simulink model "sampleModel1534"  (R2023a)
settings: Solver=VariableStepAuto  StartTime=0.0  StopTime=10.0  RelTol=1e-3
libraries: hdlsllib x7, simulink x1
settings Model: Creator=user1  LastModifiedBy=user1

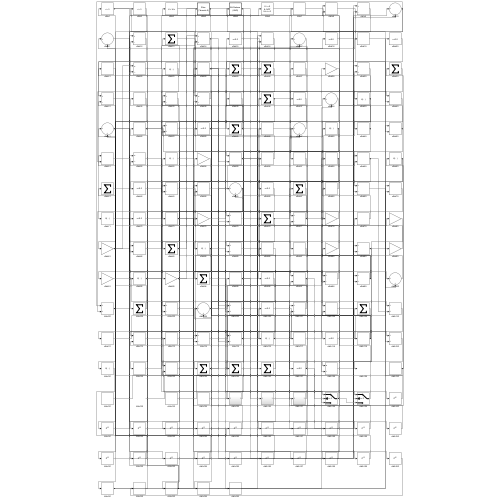
[thumbnail: Simulink's stored preview of the top-level diagram]
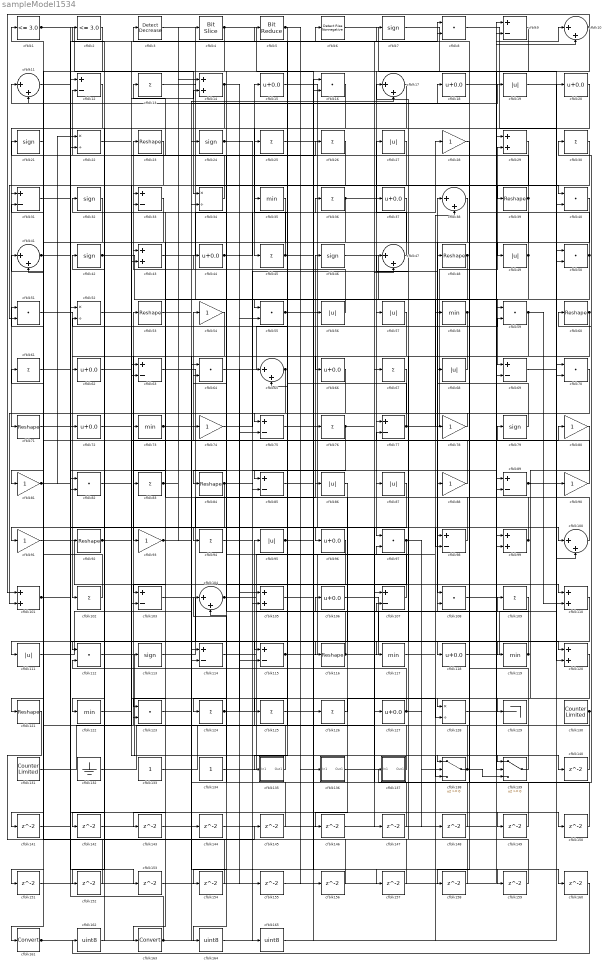
== system sampleModel1534 ==
  cfblk1 : hdlsllib/Logic and Bit Operations/Compare To Constant  relop=<=  const=3.0  OutDataTypeStr=boolean
  cfblk{10..11,17,38,41,47,65,100,104} (9 alike) : Sum  Inputs=|++
  cfblk{14,29,43,99,101,105,110,120} (8 alike) : Sum
  cfblk{13,25..26,30,36,45,61,67,76,83,94,102,109,124..126} (16 alike) : Sum  Inputs=+
  cfblk{9,12,31,33,63,69,75,77,85,89,98,103,107,114..115} (15 alike) : Sum  Inputs=+-
  cfblk{15,18,20,37,44,62,66,72,96,106,118,127} (12 alike) : Bias  Bias=0.0  SaturateOnIntegerOverflow=off
  cfblk{8,16,40,50..51,55,59,64,70,82,97,108,112,123} (14 alike) : DotProduct  OutDataTypeStr=Inherit: Inherit via internal rule
  cfblk{19,27,49,56..57,68,86..87,95,111} (10 alike) : Abs  SaturateOnIntegerOverflow=off
  cfblk{7,21,24,32,42,46,79,113} (8 alike) : Signum
  cfblk{23,39,48,53,60,71,84,92,116,121} (10 alike) : Reshape
  cfblk{35,58,73,117,119,122} (6 alike) : MinMax
  cfblk{22,34,52,128} (4 alike) : Product  Inputs=*/  RndMeth=Zero  SaturateOnIntegerOverflow=on
  cfblk129 : Terminator
  cfblk130 : hdlsllib/Sources/Counter Limited  uplimit=7  tsamp=-1
  cfblk131 : hdlsllib/Sources/Counter Limited  uplimit=7  tsamp=-1
  cfblk132 : Ground
  cfblk133 : Constant  SampleTime=-1
  cfblk134 : Constant  SampleTime=-1
  cfblk135 : Subsystem
      settings: LibrarySourceBlock=|
      | hdlsllib/Ports &
      | Subsystems/Subsystem
  cfblk136 : Subsystem
      settings: LibrarySourceBlock=|
      | hdlsllib/Ports &
      | Subsystems/Subsystem
  cfblk137 : Subsystem
      settings: LibrarySourceBlock=|
      | hdlsllib/Ports &
      | Subsystems/Subsystem
  cfblk138 : Switch  SaturateOnIntegerOverflow=off  InputSameDT=off
  cfblk139 : Switch  SaturateOnIntegerOverflow=off  InputSameDT=off
  cfblk{140..160} (21 alike) : Delay  SampleTime=1
  cfblk161 : DataTypeConversion  SaturateOnIntegerOverflow=off  RndMeth=Floor
  cfblk162 : DataTypeConversion  OutDataTypeStr=uint8  SaturateOnIntegerOverflow=off  RndMeth=Floor
  cfblk163 : DataTypeConversion  SaturateOnIntegerOverflow=off  RndMeth=Floor
  cfblk164 : DataTypeConversion  OutDataTypeStr=uint8  SaturateOnIntegerOverflow=off  RndMeth=Floor
  cfblk165 : DataTypeConversion  OutDataTypeStr=uint8  SaturateOnIntegerOverflow=off  RndMeth=Floor
  cfblk2 : hdlsllib/Logic and Bit Operations/Compare To Constant  relop=<=  const=3.0  OutDataTypeStr=boolean
  cfblk{28,54,74,78,80..81,88,90..91,93} (10 alike) : Gain
  cfblk3 : simulink/Logic and Bit Operations/Detect Decrease  vinit=0.0  OutDataTypeStr=boolean
      settings: LibrarySourceBlock=|
      | hdlsllib/Logic and Bit
      | Operations/Detect
      | Decrease
  cfblk4 : hdlsllib/Logic and Bit Operations/Bit Slice  lidx=7  ridx=0
  cfblk5 : hdlsllib/Logic and Bit Operations/Bit Reduce  mode=AND
  cfblk6 : hdlsllib/Logic and Bit Operations/Detect Rise Nonnegative  vinit=0  OutDataTypeStr=boolean
  wires:
  cfblk119/1 -> cfblk38/1, cfblk33/2, cfblk21/1
  cfblk63/1 -> cfblk96/1
  cfblk86/1 -> cfblk111/1
  cfblk14/1 -> cfblk71/1, cfblk115/2
  cfblk49/1 -> cfblk3/1, cfblk135/1(In1)
  cfblk10/1 -> cfblk101/1, cfblk22/2, cfblk154/1
  cfblk137/1(Out1) -> cfblk51/1
  cfblk17/1 -> cfblk45/1
  cfblk25/1 -> cfblk40/1
  cfblk88/1 -> cfblk54/1
  cfblk106/1 -> cfblk118/1
  cfblk39/1 -> cfblk108/1, cfblk13/1, cfblk103/2
  cfblk90/1 -> cfblk61/1
  cfblk78/1 -> cfblk75/1
  cfblk132/1 -> cfblk95/1
  cfblk70/1 -> cfblk163/1
  cfblk9/1 -> cfblk97/1
  cfblk66/1 -> cfblk101/2
  cfblk27/1 -> cfblk57/1
  cfblk15/1 -> cfblk127/1
  cfblk84/1 -> cfblk64/2, cfblk141/1, cfblk159/1
  cfblk114/1 -> cfblk109/1
  cfblk38/1 -> cfblk84/1
  cfblk60/1 -> cfblk102/1, cfblk117/1
  cfblk21/1 -> cfblk81/1
  cfblk55/1 -> cfblk98/1, cfblk89/2
  cfblk13/1 -> cfblk69/1
  cfblk89/1 -> cfblk128/1, cfblk100/2
  cfblk108/1 -> cfblk120/1
  cfblk136/1(Out1) -> cfblk30/1
  cfblk99/1 -> cfblk17/1, cfblk33/1, cfblk65/2
  cfblk45/1 -> cfblk15/1, cfblk149/1
  cfblk32/1 -> cfblk91/1
  cfblk34/1 -> cfblk12/2
  cfblk1/1 -> cfblk34/1, cfblk100/1
  cfblk36/1 -> cfblk121/1, cfblk8/1
  cfblk74/1 -> cfblk48/1
  cfblk53/1 -> cfblk17/2
  cfblk135/1(Out1) -> cfblk53/1
  cfblk113/1 -> cfblk46/1
  cfblk77/1 -> cfblk29/2, cfblk52/2
  cfblk101/1 -> cfblk41/1, cfblk153/1
  cfblk54/1 -> cfblk93/1
  cfblk59/1 -> cfblk77/1, cfblk110/2
  cfblk44/1 -> cfblk36/1, cfblk55/2
  cfblk30/1 -> cfblk69/2
  cfblk115/1 -> cfblk67/1, cfblk35/1
  cfblk43/1 -> cfblk28/1
  cfblk67/1 -> cfblk85/1
  cfblk134/1 -> cfblk106/1
  cfblk56/1 -> cfblk23/1
  cfblk127/1 -> cfblk112/2, cfblk148/1
  cfblk124/1 -> cfblk76/1, cfblk65/1
  cfblk109/1 -> cfblk107/2
  cfblk104/1 -> cfblk38/2, cfblk75/2
  cfblk3/1 -> cfblk39/1
  cfblk107/1 -> cfblk44/1
  cfblk8/1 -> cfblk40/2
  cfblk102/1 -> cfblk41/2
  cfblk52/1 -> cfblk128/2
  cfblk48/1 -> cfblk83/1, cfblk55/1
  cfblk19/1 -> cfblk90/1
  cfblk41/1 -> cfblk99/2, cfblk150/1
  cfblk83/1 -> cfblk43/1, cfblk14/1
  cfblk69/1 -> cfblk120/2
  cfblk79/1 -> cfblk68/1
  cfblk16/1 -> cfblk122/1
  cfblk5/1 -> cfblk125/1, cfblk156/1
  cfblk51/1 -> cfblk62/1
  cfblk117/1 -> cfblk79/1
  cfblk37/1 -> cfblk73/1
  cfblk47/1 -> cfblk27/1
  cfblk72/1 -> cfblk26/1
  cfblk111/1 -> cfblk18/1
  cfblk125/1 -> cfblk16/1
  cfblk42/1 -> cfblk85/2, cfblk14/2
  cfblk112/1 -> cfblk139/1
  cfblk95/1 -> cfblk19/1, cfblk136/1(In1)
  cfblk82/1 -> cfblk43/2
  cfblk118/1 -> cfblk20/1
  cfblk92/1 -> cfblk116/1, cfblk138/1
  cfblk85/1 -> cfblk16/2
  cfblk40/1 -> cfblk49/1
  cfblk65/1 -> cfblk103/1, cfblk152/1
  cfblk73/1 -> cfblk98/2, cfblk160/1
  cfblk58/1 -> cfblk123/1, cfblk114/2
  cfblk130/1 -> cfblk123/2, cfblk60/1
  cfblk26/1 -> cfblk51/2
  cfblk24/1 -> cfblk138/3, cfblk105/1, cfblk155/1
  cfblk6/1 -> cfblk139/2
  cfblk91/1 -> cfblk137/1(In1)
  cfblk138/1 -> cfblk139/3, cfblk5/1
  cfblk139/1 -> cfblk108/2
  cfblk131/1 -> cfblk63/1
  cfblk76/1 -> cfblk37/1, cfblk105/2
  cfblk2/1 -> cfblk161/1
  cfblk46/1 -> cfblk78/1
  cfblk20/1 -> cfblk25/1
  cfblk80/1 -> cfblk129/1
  cfblk50/1 -> cfblk11/2, cfblk115/1
  cfblk126/1 -> cfblk86/1
  cfblk81/1 -> cfblk72/1, cfblk22/1
  cfblk18/1 -> cfblk10/1
  cfblk87/1 -> cfblk94/1
  cfblk100/1 -> cfblk88/1
  cfblk116/1 -> cfblk32/1, cfblk9/2
  cfblk98/1 -> cfblk47/1
  cfblk94/1 -> cfblk110/1
  cfblk68/1 -> cfblk66/1
  cfblk128/1 -> cfblk10/2
  cfblk93/1 -> cfblk24/1, cfblk4/1
  cfblk57/1 -> cfblk112/1
  cfblk22/1 -> cfblk6/1
  cfblk61/1 -> cfblk119/1
  cfblk4/1 -> cfblk126/1, cfblk82/2
  cfblk23/1 -> cfblk63/2
  cfblk97/1 -> cfblk104/2, cfblk138/2
  cfblk62/1 -> cfblk113/1
  cfblk11/1 -> cfblk92/1
  cfblk133/1 -> cfblk47/2
  cfblk122/1 -> cfblk80/1
  cfblk71/1 -> cfblk87/1
  cfblk96/1 -> cfblk124/1
  cfblk7/1 -> cfblk50/2
  cfblk12/1 -> cfblk31/1
  cfblk31/1 -> cfblk7/1
  cfblk64/1 -> cfblk59/2
  cfblk75/1 -> cfblk140/1
  cfblk140/1 -> cfblk50/1
  cfblk141/1 -> cfblk12/1
  cfblk110/1 -> cfblk142/1
  cfblk142/1 -> cfblk34/2
  cfblk35/1 -> cfblk143/1
  cfblk143/1 -> cfblk29/1
  cfblk123/1 -> cfblk144/1
  cfblk121/1 -> cfblk145/1
  cfblk145/1 -> cfblk64/1
  cfblk120/1 -> cfblk146/1
  cfblk146/1 -> cfblk9/1
  cfblk103/1 -> cfblk147/1
  cfblk147/1 -> cfblk104/1
  cfblk148/1 -> cfblk107/1
  cfblk149/1 -> cfblk8/2
  cfblk150/1 -> cfblk77/2
  cfblk33/1 -> cfblk151/1
  cfblk151/1 -> cfblk99/1
  cfblk152/1 -> cfblk1/1
  cfblk153/1 -> cfblk89/1
  cfblk154/1 -> cfblk31/2
  cfblk155/1 -> cfblk59/1
  cfblk156/1 -> cfblk11/1
  cfblk105/1 -> cfblk157/1
  cfblk157/1 -> cfblk114/1
  cfblk28/1 -> cfblk158/1
  cfblk158/1 -> cfblk82/1
  cfblk159/1 -> cfblk97/2
  cfblk161/1 -> cfblk74/1, cfblk56/1
  cfblk160/1 -> cfblk162/1
  cfblk162/1 -> cfblk2/1
  cfblk163/1 -> cfblk52/1, cfblk58/1, cfblk42/1
  cfblk29/1 -> cfblk164/1
  cfblk164/1 -> cfblk70/1
  cfblk144/1 -> cfblk165/1
  cfblk165/1 -> cfblk70/2

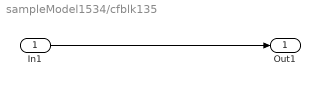
== system sampleModel1534/cfblk135 ==
  In1 : Inport
  Out1 : Outport
  wires:
  In1/1 -> Out1/1

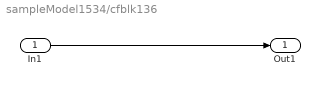
== system sampleModel1534/cfblk136 ==
  In1 : Inport
  Out1 : Outport
  wires:
  In1/1 -> Out1/1

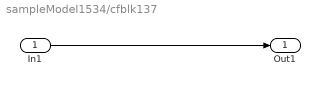
== system sampleModel1534/cfblk137 ==
  In1 : Inport
  Out1 : Outport
  wires:
  In1/1 -> Out1/1
